simulink model "Dugoff0407"  (R2019a)
settings: Solver=VariableStepAuto  StartTime=0.0  StopTime=20  RelTol=1e-3
values from neighbouring files (symbols this model uses):
  a = 1.015    [Dugoff_parameter.m]
  b = 1.895    [Dugoff_parameter.m]
  g = 9.81    [Dugoff_parameter.m]
  hg = 0.54    [Dugoff_parameter.m]
  L = a+b    (= 2.91)    [Dugoff_parameter.m]
  ms = 1270    [Dugoff_parameter.m]
  mu = 0.85    [Dugoff_parameter.m]
  mw = 35.5    [Dugoff_parameter.m]
  R = 0.325    [Dugoff_parameter.m]
  tw1 = 1.675    [Dugoff_parameter.m]
  tw2 = 1.675    [Dugoff_parameter.m]
undefined symbols (not defined in the file or in its folder): Data, Data_SL_Info
libraries: robotlib x4, Solver_SF x1, sharedTrackingLibrary x1
settings Model: Creator=qidengliang  LastModifiedBy=Administrator
settings DataIOCC: ReturnWorkspaceOutputs=off
settings DebuggingCC: ArithmeticOperatorsInVariantConditions=warning
settings SFSimCC: SimUseLocalCustomCode=off
settings RTWCC: RTWUseLocalCustomCode=off

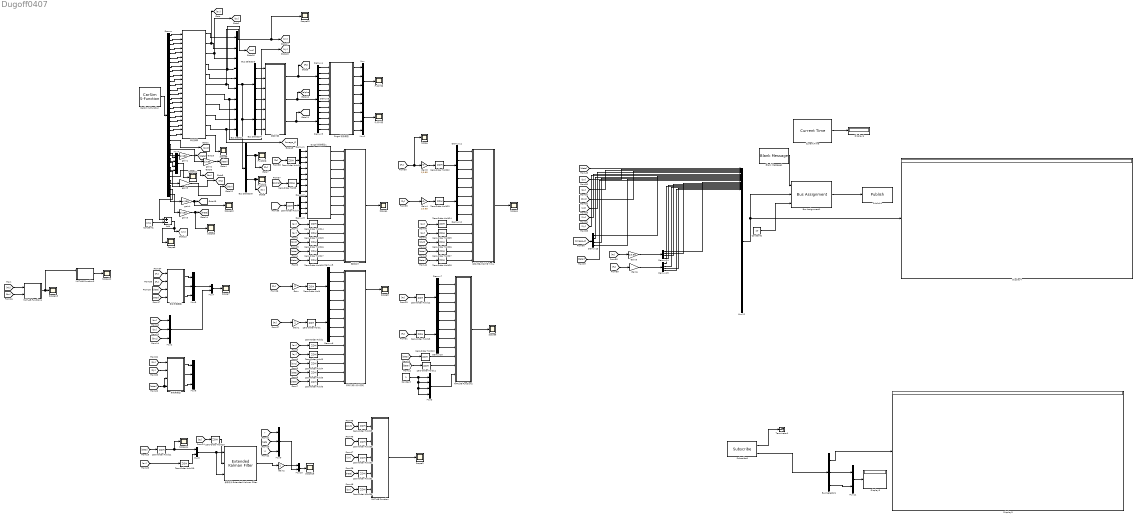
== system Dugoff0407 ==
  Add : Sum  Inputs=+-
  Blank Message1 : robotlib/Blank Message  messageClass=Message  entityType=std_msgs/Float64MultiArray  messageType=std_msgs/Float64MultiArray  SampleTime=-1
      settings: SourceProductBaseCode=RO
  Bus Assignment1 : BusAssignment  AssignedSignals=Data,Data_SL_Info.CurrentLength
  Bus Creator : BusCreator  Inputs=10
  Bus Selector1 : BusSelector  OutputSignals=Data,Data_SL_Info.CurrentLength,Data_SL_Info.ReceivedLength
  Bus Selector3 : BusSelector  OutputSignals=delta,ax,ay,omega
  Bus Selector4 : BusSelector  OutputSignals=Vx,Vy,r
  Bus Selector5 : BusSelector  OutputSignals=Fx,Fy
  CarSim S-Function : Solver_SF/CarSim S-Function  Priority=1  SIMFILE=simfile.sim
  Constant : Constant
  Constant1 : Constant  Value=0.54
  Constant2 : Constant  Value=20  OutDataTypeStr=uint32
  Current Time : robotlib/Current Time  OutputFormat=double  SampleTime=-1  ModelName=Dugoff0407
      settings: SourceProductName=Robotics System Toolbox  SourceProductBaseCode=RO
  Demux : Demux  Outputs=36
  Demux{1..15} (15 alike) : Demux
  Display{3..6} (4 alike) : Display
      Display3 settings: Format=long_e  Decimation=5
      Display4 settings: Format=long_e  Decimation=5
  Dugoff轮胎模型 : Subsystem
  Dugoff轮胎模型1 : Subsystem
  Fx估计值 : Scope
  Fx实际值 : Scope
  Fy估计值 : Scope
  Fy实际值 : Scope
  Gain : Gain  Gain=2
  Gain1 : Gain  Gain=2
  Gain2 : Gain
  Gain{3..6} (4 alike) : Gain  Gain=1/0.85
  MATLAB Function : MATLAB Function  TreatAsAtomicUnit=on
  MATLAB Function2 : MATLAB Function  TreatAsAtomicUnit=on
  MATLAB Function3 : MATLAB Function  TreatAsAtomicUnit=on
  MATLAB Function4 : MATLAB Function  TreatAsAtomicUnit=on
  Mux{,1,3..4} (4 alike) : Mux
  Mux{7..8,10..11} (4 alike) : Mux  Inputs=2
  Mux12 : Mux  Inputs=128
  Mux{2,5..6,9} (4 alike) : Mux  Inputs=3
  Publish1 : robotlib/Publish  topicSource=Specify your own  topic=/chatter/matlab  messageType=std_msgs/Float64MultiArray  messageQueueLength=1
      settings: SourceProductBaseCode=RO
  Scope{,1..16} (17 alike) : Scope
  Subscribe1 : robotlib/Subscribe  topicSource=Select from ROS network  topic=/chatter/array0  messageType=std_msgs/Float64MultiArray  sampleTime=-1  messageQueueLength=1
      settings: SourceProductBaseCode=RO
  Terminator1 : Terminator
  Zero-Order Hold{,1..33} (34 alike) : ZeroOrderHold  SampleTime=0.01
  gain{1..4} (4 alike) : Gain  Gain=pi/180
  gain5 : Gain  Gain=9.80665
  修正车辆模型 : MATLAB Function  TreatAsAtomicUnit=on
  单位换算 : Subsystem
  单转角模型 : MATLAB Function  TreatAsAtomicUnit=on
  参数估计Extended Kalman Filter : sharedTrackingLibrary/Extended Kalman Filter  StateTransitionFcn=LinearState2_u  HasStateTransitionJacobianFcn=off  HasAdditiveProcessNoise=Additive  ProcessNoise=diag([1 1 1])  HasTimeVaryingProcessNoise=off  HasStateTransitionFcnExtraArgument=1  InitialState=[0,0,13.9]  InitialStateCovariance=0.1  MeasurementFcn1=Sensor_ax_u2  HasMeasurementJacobianFcn1=off  HasMeasurementEnablePort1=off  HasAdditiveMeasurementNoise1=Additive  MeasurementNoise1=50  HasTimeVaryingMeasurementNoise1=off  HasMeasurementFcnExtraArgument1=1  MeasurementFcn2=myMeasurementFcn  HasMeasurementJacobianFcn2=off  HasMeasurementEnablePort2=off  HasAdditiveMeasurementNoise2=Additive  MeasurementNoise2=1  HasTimeVaryingMeasurementNoise2=off  HasMeasurementFcnExtraArgument2=0  MeasurementFcn3=myMeasurementFcn  HasMeasurementJacobianFcn3=off  HasMeasurementEnablePort3=off  HasAdditiveMeasurementNoise3=Additive  MeasurementNoise3=1  HasTimeVaryingMeasurementNoise3=off  HasMeasurementFcnExtraArgument3=0  MeasurementFcn4=myMeasurementFcn  HasMeasurementJacobianFcn4=off  HasMeasurementEnablePort4=off  HasAdditiveMeasurementNoise4=Additive  MeasurementNoise4=1  HasTimeVaryingMeasurementNoise4=off  HasMeasurementFcnExtraArgument4=0  MeasurementFcn5=myMeasurementFcn  HasMeasurementJacobianFcn5=off  HasMeasurementEnablePort5=off  HasAdditiveMeasurementNoise5=Additive  MeasurementNoise5=1  HasTimeVaryingMeasurementNoise5=off  HasMeasurementFcnExtraArgument5=0  EnableMultirate=off  StateTransitionFcnSampleTime=1  MeasurementFcn1SampleTime=1  MeasurementFcn2SampleTime=1  MeasurementFcn3SampleTime=1  MeasurementFcn4SampleTime=1  MeasurementFcn5SampleTime=1  UseCurrentEstimator=on  OutputStateCovariance=off  DataType=double  SampleTime=0.01  NumberOfMeasurements=1
      settings: SourceProductBaseCode=CT,DR,TF,ID,LP,NV,AR,RO,RR,UV,VE
  参数计算 : Subsystem
  实际力输入估计单个miu : MATLAB Function  TreatAsAtomicUnit=on
  实际力输入估计四轮 : MATLAB Function  TreatAsAtomicUnit=on
  整体估计 : MATLAB Function  TreatAsAtomicUnit=on
  wires:
  Demux/5 -> 单位换算/5(In5)
  Bus Selector5/1 -> [Fx], Fx实际值/1  "<Fx>"
  Demux/2 -> 单位换算/2(In2)
  Bus Selector3/2 -> 参数计算/2(ax)  "<ax>"
  CarSim S-Function/1 -> Demux/1
  Demux/23 -> 单位换算/23(In23)
  单位换算/11(alpha) -> Scope9/1  "真实值"
  单位换算/6(纵向车速) -> Scope15/1, [Vx], Bus Creator/6  "Vx"
  Demux/16 -> 单位换算/16(In16)
  Bus Creator/1 -> Bus Selector5/1, Bus Selector4/1, Bus Selector3/1
  Demux/22 -> 单位换算/22(In22)
  Demux/20 -> 单位换算/20(In20)
  Demux/12 -> 单位换算/12(In12)
  Demux/7 -> 单位换算/7(In7)
  Demux/21 -> 单位换算/21(In21)
  Demux/14 -> 单位换算/14(In14)
  Demux/9 -> 单位换算/9(In9)
  Demux/11 -> 单位换算/11(In11)
  Bus Selector5/2 -> [Fy], Fy实际值/1  "<Fy>"
  Bus Selector4/3 -> 参数计算/7(r)  "<r>"
  单位换算/4(横摆角速度) -> [wz], Bus Creator/4  "r"
  单位换算/3(侧向加速度) -> Bus Creator/3, [ay]  "ay"
  Demux4/3 -> Dugoff轮胎模型/3(Fz21)
  Demux/15 -> 单位换算/15(In15)
  单位换算/9(Fy_ij) -> Bus Creator/9  "Fy"
  Demux/1 -> 单位换算/1(In1)
  Demux/17 -> 单位换算/17(In17)
  单位换算/10(Omega_ij) -> [omega_ij], Bus Creator/10  "omega"
  单位换算/5(质心侧偏角) -> Bus Creator/5  "beta"
  Demux8/4 -> Dugoff轮胎模型/8(alpha22)
  Demux8/2 -> Dugoff轮胎模型/6(alpha12)
  Demux/8 -> 单位换算/8(In8)
  Bus Selector3/1 -> 参数计算/1(delta)  "<delta>"
  Demux/10 -> 单位换算/10(In10)
  Demux9/1 -> Dugoff轮胎模型/9(lamda11)
  Demux4/2 -> Dugoff轮胎模型/2(Fz12)
  Demux/18 -> 单位换算/18(In18)
  Demux/6 -> 单位换算/6(In6)
  单位换算/7(侧向车速) -> [Vy], Bus Creator/7  "Vy"
  Demux4/4 -> Dugoff轮胎模型/4(Fz22)
  Demux9/2 -> Dugoff轮胎模型/10(lamda12)
  Demux9/3 -> Dugoff轮胎模型/11(lamda21)
  Bus Selector3/3 -> 参数计算/3(ay)  "<ay>"
  Demux4/1 -> Dugoff轮胎模型/1(Fz11)
  Demux/13 -> 单位换算/13(In13)
  Demux9/4 -> Dugoff轮胎模型/12(lamda22)
  单位换算/2(纵向加速度) -> Bus Creator/2, [ax]  "ax"
  Demux8/3 -> Dugoff轮胎模型/7(alpha21)
  单位换算/8(Fx_ij) -> Bus Creator/8  "Fx"
  Demux8/1 -> Dugoff轮胎模型/5(alpha11)
  Bus Selector4/2 -> 参数计算/6(Vy)  "<Vy>"
  Demux/4 -> 单位换算/4(In4)
  Demux/19 -> 单位换算/19(In19)
  单位换算/1(前轮转角) -> Bus Creator/1  "delta"
  Bus Selector4/1 -> 参数计算/5(Vx)  "<Vx>"
  Demux/3 -> 单位换算/3(In3)
  Bus Selector3/4 -> 参数计算/4(omega)  "<omega>"
  Dugoff轮胎模型/3(Fx21) -> Mux/3
  Dugoff轮胎模型/2(Fx12) -> Mux/2
  Dugoff轮胎模型/1(Fx11) -> Mux/1
  Dugoff轮胎模型/4(Fx22) -> Mux/4
  Dugoff轮胎模型/5(Fy11) -> Mux1/1
  Dugoff轮胎模型/6(Fy12) -> Mux1/2
  Dugoff轮胎模型/7(Fy21) -> Mux1/3
  Dugoff轮胎模型/8(Fy22) -> Mux1/4
  Mux1/1 -> Fy估计值/1
  Mux/1 -> Fx估计值/1
  参数计算/1(Fz) -> [Fz], Demux4/1  "计算值"
  Demux1/1 -> Dugoff轮胎模型1/1(Fz11)
  Demux1/4 -> Dugoff轮胎模型1/4(Fz22)
  Demux1/2 -> Dugoff轮胎模型1/2(Fz12)
  Demux1/3 -> Dugoff轮胎模型1/3(Fz21)
  参数计算/2(alpha) -> [alpha], Demux8/1  "计算值"
  Demux2/1 -> Dugoff轮胎模型1/5(alpha11)
  Demux2/3 -> Dugoff轮胎模型1/7(alpha21)
  Demux3/4 -> Dugoff轮胎模型1/12(lamda22)
  Demux3/3 -> Dugoff轮胎模型1/11(lamda21)
  Demux3/2 -> Dugoff轮胎模型1/10(lamda12)
  Demux3/1 -> Dugoff轮胎模型1/9(lamda11)
  Demux2/2 -> Dugoff轮胎模型1/6(alpha12)
  Demux2/4 -> Dugoff轮胎模型1/8(alpha22)
  参数计算/3(lamda) -> [lamda], Demux9/1
  Dugoff轮胎模型1/8(Fy22) -> 整体估计/8(Fyrr)
  Dugoff轮胎模型1/7(Fy21) -> 整体估计/7(Fyrl)
  Dugoff轮胎模型1/6(Fy12) -> 整体估计/6(Fyfr)
  Dugoff轮胎模型1/5(Fy11) -> 整体估计/5(Fyfl)
  Dugoff轮胎模型1/4(Fx22) -> 整体估计/4(Fxrr)
  Dugoff轮胎模型1/3(Fx21) -> 整体估计/3(Fxrl)
  Dugoff轮胎模型1/2(Fx12) -> 整体估计/2(Fxfr)
  Dugoff轮胎模型1/1(Fx11) -> 整体估计/1(Fxfl)
  整体估计/1(x0) -> Scope4/1
  Demux/24 -> [dwz]
  gain1/1 -> [deta]
  Demux/25 -> gain1/1
  gain2/1 -> [detar]
  Demux/26 -> gain2/1
  实际力输入估计四轮/1(x0) -> Scope5/1
  Demux5/1 -> 实际力输入估计四轮/1(Fxfl)
  Demux5/2 -> 实际力输入估计四轮/2(Fxfr)
  Demux5/3 -> 实际力输入估计四轮/3(Fxrl)
  Demux5/4 -> 实际力输入估计四轮/4(Fxrr)
  Demux6/1 -> 实际力输入估计四轮/5(Fyfl)
  Demux6/2 -> 实际力输入估计四轮/6(Fyfr)
  Demux6/3 -> 实际力输入估计四轮/7(Fyrl)
  Demux6/4 -> 实际力输入估计四轮/8(Fyrr)
  Gain/1 -> Zero-Order Hold/1
  Gain1/1 -> Zero-Order Hold1/1
  Zero-Order Hold2/1 -> 实际力输入估计四轮/9(ax)
  Zero-Order Hold3/1 -> 实际力输入估计四轮/10(ay)
  Zero-Order Hold4/1 -> 实际力输入估计四轮/11(dwz)
  Zero-Order Hold5/1 -> 实际力输入估计四轮/12(deta)
  Zero-Order Hold6/1 -> 实际力输入估计四轮/13(detar)
  [detar] -> Zero-Order Hold6/1
  [deta] -> Zero-Order Hold5/1
  [ay] -> Zero-Order Hold3/1
  [dwz] -> Zero-Order Hold4/1
  [ax] -> Zero-Order Hold2/1
  [deta] -> Zero-Order Hold10/1
  [detar] -> Zero-Order Hold11/1
  Zero-Order Hold11/1 -> MATLAB Function2/10(detar)
  Zero-Order Hold10/1 -> MATLAB Function2/9(deta)
  Zero-Order Hold13/1 -> Demux10/1
  Zero-Order Hold12/1 -> Demux7/1
  Demux10/4 -> MATLAB Function2/8(Fyrr)
  Demux10/3 -> MATLAB Function2/7(Fyrl)
  Demux10/2 -> MATLAB Function2/6(Fyfr)
  Demux10/1 -> MATLAB Function2/5(Fyfl)
  Demux7/4 -> MATLAB Function2/4(Fxrr)
  Demux7/3 -> MATLAB Function2/3(Fxrl)
  Demux7/2 -> MATLAB Function2/2(Fxfr)
  Zero-Order Hold1/1 -> Demux6/1  "<Fy>"
  Zero-Order Hold/1 -> Demux5/1  "<Fx>"
  MATLAB Function2/1(zjian) -> Scope6/1
  [ax] -> Mux2/1
  [dwz] -> Mux2/3
  [ay] -> Mux2/2
  Constant/1 -> Mux3/4, Mux3/3, Mux3/2, Mux3/1
  Mux3/1 -> MATLAB Function2/11(x0)
  Zero-Order Hold7/1 -> Demux3/1
  Zero-Order Hold8/1 -> Demux2/1
  Zero-Order Hold9/1 -> Demux1/1
  [ax] -> Zero-Order Hold14/1
  [dwz] -> Zero-Order Hold16/1
  [ay] -> Zero-Order Hold15/1
  [deta] -> Zero-Order Hold17/1
  [detar] -> Zero-Order Hold18/1
  Zero-Order Hold18/1 -> 整体估计/13(detar)
  Zero-Order Hold17/1 -> 整体估计/12(deta)
  Zero-Order Hold16/1 -> 整体估计/11(dwz)
  Zero-Order Hold15/1 -> 整体估计/10(ay)
  Zero-Order Hold14/1 -> 整体估计/9(ax)
  Demux/27 -> Mux4/1
  Demux/28 -> Mux4/2
  Demux/29 -> Mux4/3
  Demux/30 -> Mux4/4
  Mux4/1 -> Scope11/1
  MATLAB Function3/1(y) -> Scope12/1
  Demux7/1 -> MATLAB Function2/1(Fxfl)
  Demux/31 -> [Tb]
  Demux/32 -> [dw]
  [Tb] -> MATLAB Function4/1(Tb)
  [dw] -> MATLAB Function4/2(dw)
  MATLAB Function4/1(y) -> MATLAB Function3/1(Fx), Scope13/1
  [deta] -> 修正车辆模型/3(detal)
  [detar] -> 修正车辆模型/4(detar)
  修正车辆模型/1(ax) -> Mux5/1
  修正车辆模型/3(dwz) -> Mux5/3
  [deta] -> 单转角模型/3(detal), 单转角模型/4(detar)
  单转角模型/3(dwz) -> Mux6/3
  单转角模型/2(ay) -> Mux6/2
  单转角模型/1(ax) -> Mux6/1
  修正车辆模型/2(ay) -> Mux5/2
  参数估计Extended Kalman Filter/1 -> Gain2/1
  Mux8/1 -> 参数估计Extended Kalman Filter/3, 参数估计Extended Kalman Filter/1
  Zero-Order Hold20/1 -> 参数估计Extended Kalman Filter/2
  Zero-Order Hold19/1 -> Mux8/2
  Zero-Order Hold21/1 -> Scope14/1, Mux8/1
  [deta] -> Zero-Order Hold21/1
  [beta] -> Mux9/2
  [r] -> Mux9/1
  [vx] -> Mux9/3
  Mux9/1 -> Mux10/2
  Gain2/1 -> Mux10/1
  Mux10/1 -> Scope16/1
  [ay] -> Zero-Order Hold20/1
  Mux5/1 -> Mux7/1
  Mux2/1 -> Mux7/2
  Mux7/1 -> Scope7/1
  [ax] -> Zero-Order Hold19/1
  [Fx] -> Gain/1
  [Fy] -> Gain1/1
  [Fx] -> Zero-Order Hold12/1
  [Fy] -> Zero-Order Hold13/1
  [Fx] -> 单转角模型/1(Fx)
  [Fy] -> 单转角模型/2(Fy)
  [Fy] -> 修正车辆模型/2(Fy)
  [Fx] -> 修正车辆模型/1(Fx)
  [lamda] -> Zero-Order Hold7/1
  [alpha] -> Zero-Order Hold8/1
  [Fz] -> Zero-Order Hold9/1
  [Fy] -> Gain4/1
  [Fx] -> Scope/1, Gain3/1
  Zero-Order Hold22/1 -> Demux11/1
  Zero-Order Hold23/1 -> Demux12/1
  [ax] -> Zero-Order Hold24/1
  [dwz] -> Zero-Order Hold26/1
  [ay] -> Zero-Order Hold25/1
  [deta] -> Zero-Order Hold27/1
  [detar] -> Zero-Order Hold28/1
  Zero-Order Hold28/1 -> 实际力输入估计单个miu/13(detar)
  Zero-Order Hold27/1 -> 实际力输入估计单个miu/12(deta)
  Zero-Order Hold26/1 -> 实际力输入估计单个miu/11(dwz)
  Zero-Order Hold25/1 -> 实际力输入估计单个miu/10(ay)
  Zero-Order Hold24/1 -> 实际力输入估计单个miu/9(ax)
  Gain4/1 -> Zero-Order Hold23/1
  Gain3/1 -> Zero-Order Hold22/1
  Demux12/4 -> 实际力输入估计单个miu/8(Fyrr)
  Demux12/3 -> 实际力输入估计单个miu/7(Fyrl)
  Demux12/2 -> 实际力输入估计单个miu/6(Fyfr)
  Demux12/1 -> 实际力输入估计单个miu/5(Fyfl)
  Demux11/4 -> 实际力输入估计单个miu/4(Fxrr)
  Demux11/3 -> 实际力输入估计单个miu/3(Fxrl)
  Demux11/2 -> 实际力输入估计单个miu/2(Fxfr)
  Demux11/1 -> 实际力输入估计单个miu/1(Fxfl)
  实际力输入估计单个miu/1(x0) -> Scope1/1
  gain3/1 -> Scope3/1, [theta]
  Demux/36 -> gain3/1
  Demux/34 -> gain4/1
  gain4/1 -> Scope10/1, [dtheta]
  gain5/1 -> [ddxh]
  Demux/33 -> gain5/1
  [theta] -> Zero-Order Hold32/1
  [ddxh] -> Zero-Order Hold29/1
  [dtheta] -> Zero-Order Hold30/1
  [xh] -> Zero-Order Hold31/1
  [ax] -> Zero-Order Hold33/1
  MATLAB Function/1(x0) -> Scope2/1
  Zero-Order Hold29/1 -> MATLAB Function/1(ddxh)
  Zero-Order Hold30/1 -> MATLAB Function/2(dtheta)
  Zero-Order Hold31/1 -> MATLAB Function/3(xh)
  Zero-Order Hold32/1 -> MATLAB Function/4(theta)
  Zero-Order Hold33/1 -> MATLAB Function/5(ax)
  Demux/35 -> Add/1
  Constant1/1 -> Add/2
  Add/1 -> Scope8/1, [xh]
  Demux14/4 -> Mux12/16
  Bus Selector1/1 -> Display3/1  "<Data>"
  Mux11/1 -> Display5/1
  Demux15/4 -> Mux12/20
  Subscribe1/1 -> Terminator1/1
  Gain6/1 -> Demux15/1
  [Fx] -> Gain5/1
  [Fy] -> Gain6/1
  [deta] -> Mux12/1  "delta"
  Bus Selector1/2 -> Mux11/1  "<CurrentLength>"
  Subscribe1/2 -> Bus Selector1/1
  Constant2/1 -> Bus Assignment1/3
  [wz] -> Mux12/5  "wz"
  Demux14/2 -> Mux12/14
  Demux15/1 -> Mux12/17
  Demux15/2 -> Mux12/18
  Current Time/1 -> Display6/1
  Demux15/3 -> Mux12/19
  Demux13/4 -> Mux12/11
  Demux13/2 -> Mux12/9
  Demux14/1 -> Mux12/13
  [Vy] -> Mux12/7  "Vy"
  Gain5/1 -> Demux14/1
  [detar] -> Mux12/12  "deltar"
  Bus Selector1/3 -> Mux11/2  "<ReceivedLength>"
  Demux14/3 -> Mux12/15
  [dwz] -> Mux12/4  "dwz"
  [Vx] -> Mux12/6  "Vx"
  Blank Message1/1 -> Bus Assignment1/1
  Demux13/3 -> Mux12/10
  [ax] -> Mux12/2  "ax"
  Demux13/1 -> Mux12/8
  Bus Assignment1/1 -> Publish1/1
  [omega_ij] -> Demux13/1
  Mux12/1 -> Display4/1, Bus Assignment1/2
  [ay] -> Mux12/3  "ay"

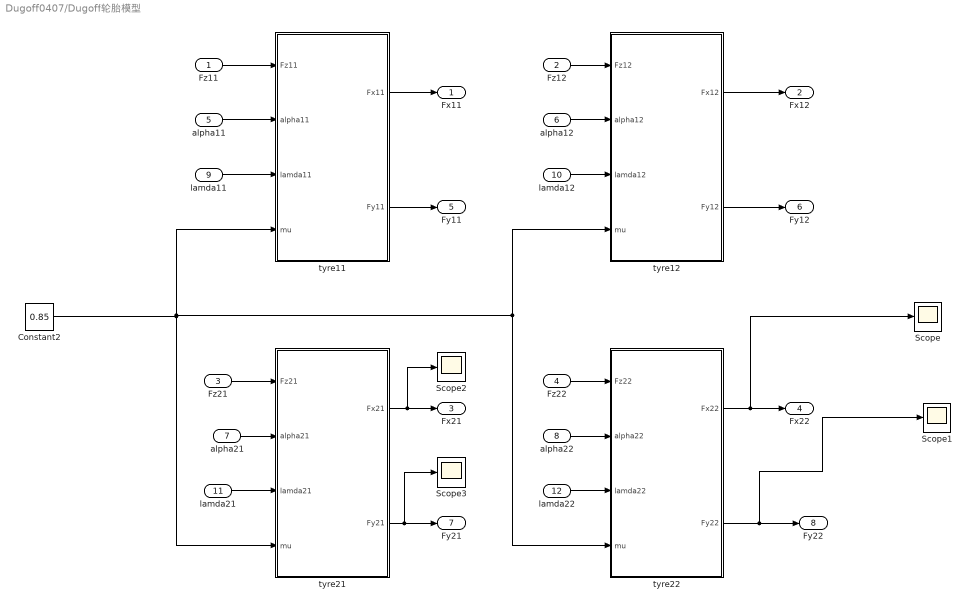
== system Dugoff0407/Dugoff轮胎模型 ==
  Fz11 : Inport
  Fz12 : Inport  Port=2
  Fz21 : Inport  Port=3
  Fz22 : Inport  Port=4
  alpha11 : Inport  Port=5
  alpha12 : Inport  Port=6
  alpha21 : Inport  Port=7
  alpha22 : Inport  Port=8
  lamda11 : Inport  Port=9
  lamda12 : Inport  Port=10
  lamda21 : Inport  Port=11
  lamda22 : Inport  Port=12
  Constant2 : Constant  Value=0.85
  Scope{,1..3} (4 alike) : Scope
  tyre11 : MATLAB Function  TreatAsAtomicUnit=on
  tyre12 : MATLAB Function  TreatAsAtomicUnit=on
  tyre21 : MATLAB Function  TreatAsAtomicUnit=on
  tyre22 : MATLAB Function  TreatAsAtomicUnit=on
  Fx11 : Outport
  Fx12 : Outport  Port=2
  Fx21 : Outport  Port=3
  Fx22 : Outport  Port=4
  Fy11 : Outport  Port=5
  Fy12 : Outport  Port=6
  Fy21 : Outport  Port=7
  Fy22 : Outport  Port=8
  wires:
  Constant2/1 -> tyre11/4(mu), tyre22/4(mu), tyre12/4(mu), tyre21/4(mu)
  alpha21/1 -> tyre21/2(alpha21)
  tyre22/2(Fy22) -> Scope1/1, Fy22/1
  Fz12/1 -> tyre12/1(Fz12)
  Fz21/1 -> tyre21/1(Fz21)
  tyre21/2(Fy21) -> Scope3/1, Fy21/1
  tyre12/2(Fy12) -> Fy12/1
  lamda12/1 -> tyre12/3(lamda12)
  tyre11/1(Fx11) -> Fx11/1
  tyre12/1(Fx12) -> Fx12/1
  tyre22/1(Fx22) -> Scope/1, Fx22/1
  lamda22/1 -> tyre22/3(lamda22)
  alpha12/1 -> tyre12/2(alpha12)
  Fz11/1 -> tyre11/1(Fz11)
  alpha11/1 -> tyre11/2(alpha11)
  lamda21/1 -> tyre21/3(lamda21)
  lamda11/1 -> tyre11/3(lamda11)
  Fz22/1 -> tyre22/1(Fz22)
  alpha22/1 -> tyre22/2(alpha22)
  tyre11/2(Fy11) -> Fy11/1
  tyre21/1(Fx21) -> Scope2/1, Fx21/1

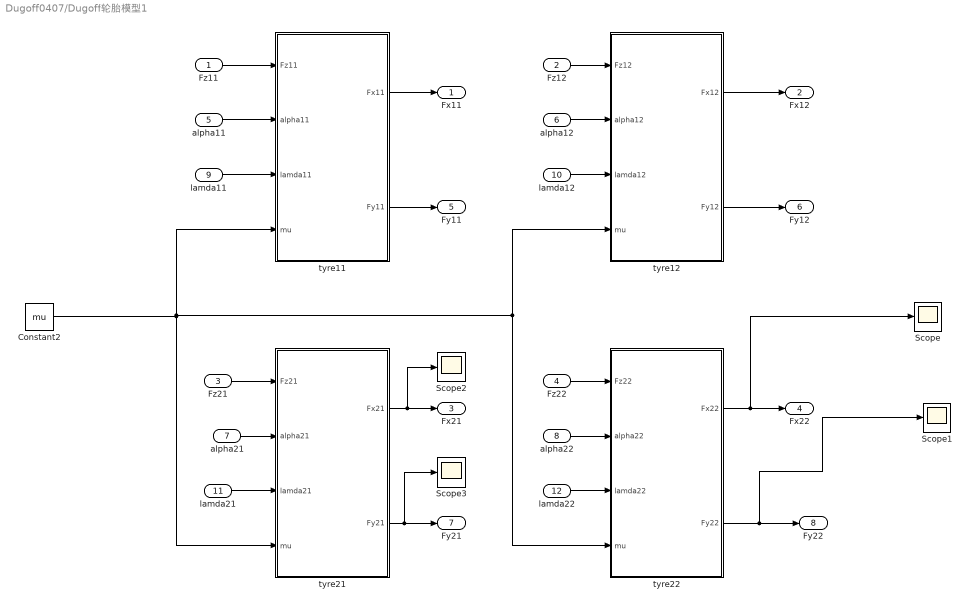
== system Dugoff0407/Dugoff轮胎模型1 ==
  Fz11 : Inport
  Fz12 : Inport  Port=2
  Fz21 : Inport  Port=3
  Fz22 : Inport  Port=4
  alpha11 : Inport  Port=5
  alpha12 : Inport  Port=6
  alpha21 : Inport  Port=7
  alpha22 : Inport  Port=8
  lamda11 : Inport  Port=9
  lamda12 : Inport  Port=10
  lamda21 : Inport  Port=11
  lamda22 : Inport  Port=12
  Constant2 : Constant  Value=mu
  Scope{,1..3} (4 alike) : Scope
  tyre11 : MATLAB Function  TreatAsAtomicUnit=on
  tyre12 : MATLAB Function  TreatAsAtomicUnit=on
  tyre21 : MATLAB Function  TreatAsAtomicUnit=on
  tyre22 : MATLAB Function  TreatAsAtomicUnit=on
  Fx11 : Outport
  Fx12 : Outport  Port=2
  Fx21 : Outport  Port=3
  Fx22 : Outport  Port=4
  Fy11 : Outport  Port=5
  Fy12 : Outport  Port=6
  Fy21 : Outport  Port=7
  Fy22 : Outport  Port=8
  wires:
  tyre21/1(Fx21) -> Fx21/1, Scope2/1
  tyre11/2(Fy11) -> Fy11/1
  alpha22/1 -> tyre22/2(alpha22)
  Fz22/1 -> tyre22/1(Fz22)
  lamda11/1 -> tyre11/3(lamda11)
  lamda21/1 -> tyre21/3(lamda21)
  alpha11/1 -> tyre11/2(alpha11)
  Fz11/1 -> tyre11/1(Fz11)
  alpha12/1 -> tyre12/2(alpha12)
  lamda22/1 -> tyre22/3(lamda22)
  tyre22/1(Fx22) -> Fx22/1, Scope/1
  tyre12/1(Fx12) -> Fx12/1
  tyre11/1(Fx11) -> Fx11/1
  lamda12/1 -> tyre12/3(lamda12)
  tyre12/2(Fy12) -> Fy12/1
  tyre21/2(Fy21) -> Fy21/1, Scope3/1
  Fz21/1 -> tyre21/1(Fz21)
  Fz12/1 -> tyre12/1(Fz12)
  tyre22/2(Fy22) -> Fy22/1, Scope1/1
  alpha21/1 -> tyre21/2(alpha21)
  Constant2/1 -> tyre21/4(mu), tyre12/4(mu), tyre22/4(mu), tyre11/4(mu)

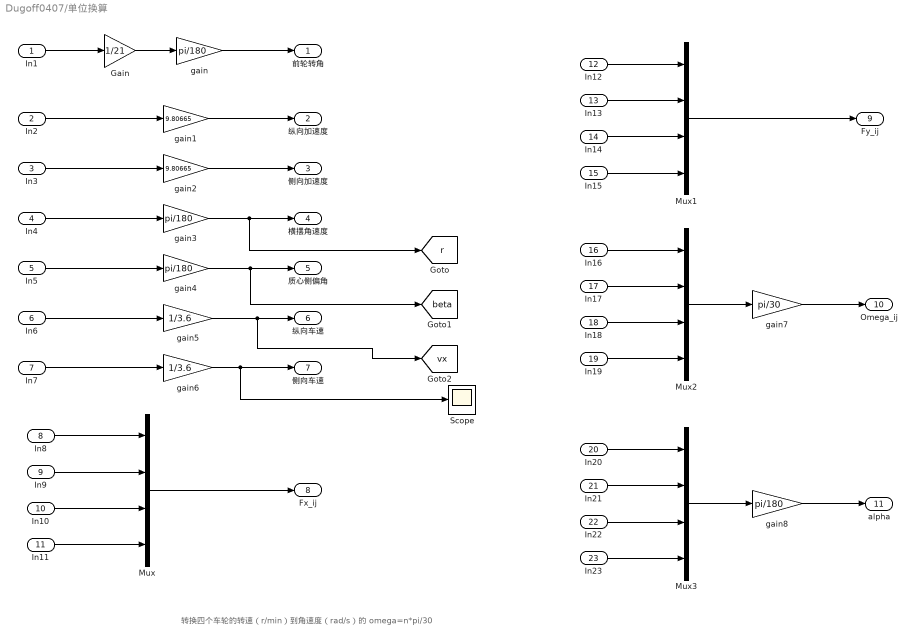
== system Dugoff0407/单位换算 ==
  note: 转换四个车轮的转速（r/min）到角速度（rad/s）的
      | omega=n*pi/30
  In1 : Inport
  In2 : Inport  Port=2
  In3 : Inport  Port=3
  In4 : Inport  Port=4
  In5 : Inport  Port=5
  In6 : Inport  Port=6
  In7 : Inport  Port=7
  In8 : Inport  Port=8
  In9 : Inport  Port=9
  In10 : Inport  Port=10
  In11 : Inport  Port=11
  In12 : Inport  Port=12
  In13 : Inport  Port=13
  In14 : Inport  Port=14
  In15 : Inport  Port=15
  In16 : Inport  Port=16
  In17 : Inport  Port=17
  In18 : Inport  Port=18
  In19 : Inport  Port=19
  In20 : Inport  Port=20
  In21 : Inport  Port=21
  In22 : Inport  Port=22
  In23 : Inport  Port=23
  Gain : Gain  Gain=1/21
  Mux{,1..3} (4 alike) : Mux
  Scope : Scope
  gain{,3..4,8} (4 alike) : Gain  Gain=pi/180
  gain1 : Gain  Gain=9.80665
  gain2 : Gain  Gain=9.80665
  gain5 : Gain  Gain=1/3.6
  gain6 : Gain  Gain=1/3.6
  gain7 : Gain  Gain=pi/30
  前轮转角 : Outport
  纵向加速度 : Outport  Port=2
  侧向加速度 : Outport  Port=3
  横摆角速度 : Outport  Port=4
  质心侧偏角 : Outport  Port=5
  纵向车速 : Outport  Port=6
  侧向车速 : Outport  Port=7
  Fx_ij : Outport  Port=8
  Fy_ij : Outport  Port=9
  Omega_ij : Outport  Port=10
  alpha : Outport  Port=11
  tag scope: beta=global, r=global, vx=global
  wires:
  In8/1 -> Mux/1
  In10/1 -> Mux/3
  In1/1 -> Gain/1
  In15/1 -> Mux1/4
  In9/1 -> Mux/2
  In11/1 -> Mux/4
  Mux/1 -> Fx_ij/1
  In14/1 -> Mux1/3
  In12/1 -> Mux1/1
  In13/1 -> Mux1/2
  gain/1 -> 前轮转角/1
  In2/1 -> gain1/1
  In3/1 -> gain2/1
  In4/1 -> gain3/1
  In5/1 -> gain4/1
  In6/1 -> gain5/1
  In7/1 -> gain6/1
  gain1/1 -> 纵向加速度/1
  gain2/1 -> 侧向加速度/1
  gain3/1 -> [r], 横摆角速度/1
  gain4/1 -> [beta], 质心侧偏角/1
  gain5/1 -> [vx], 纵向车速/1
  gain6/1 -> Scope/1, 侧向车速/1
  Gain/1 -> gain/1
  Mux1/1 -> Fy_ij/1
  gain7/1 -> Omega_ij/1
  Mux2/1 -> gain7/1
  In16/1 -> Mux2/1
  In17/1 -> Mux2/2
  In18/1 -> Mux2/3
  In19/1 -> Mux2/4
  In21/1 -> Mux3/2
  In22/1 -> Mux3/3
  In20/1 -> Mux3/1
  In23/1 -> Mux3/4
  Mux3/1 -> gain8/1
  gain8/1 -> alpha/1

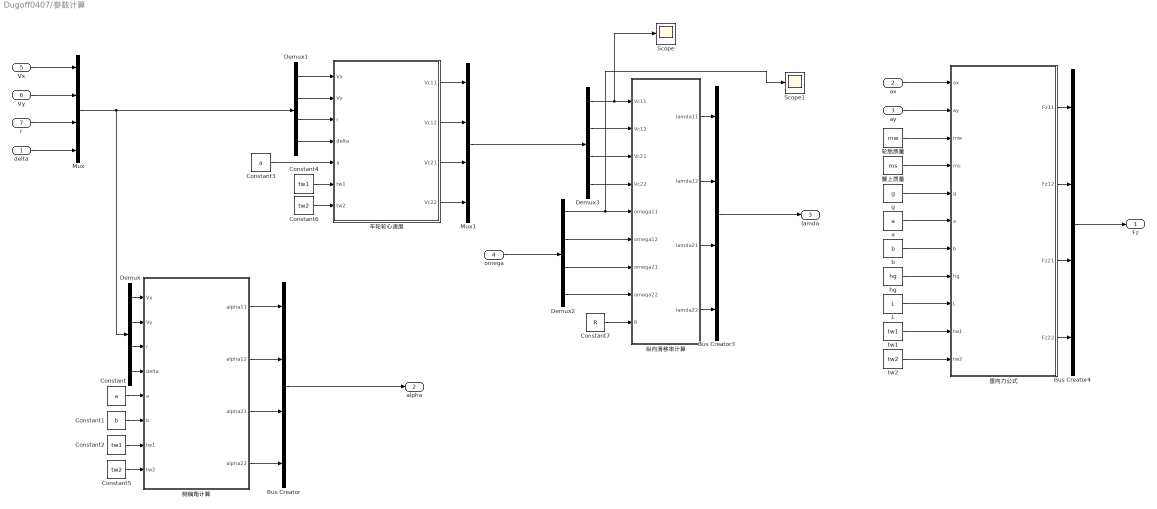
== system Dugoff0407/参数计算 ==
  delta : Inport
  ax : Inport  Port=2
  ay : Inport  Port=3
  omega : Inport  Port=4
  Vx : Inport  Port=5
  Vy : Inport  Port=6
  r : Inport  Port=7
  Bus Creator : BusCreator  Inputs=4
  Bus Creator3 : BusCreator  Inputs=4
  Bus Creator4 : BusCreator  Inputs=4
  Constant : Constant  Value=a
  Constant1 : Constant  Value=b
  Constant2 : Constant  Value=tw1
  Constant3 : Constant  Value=a
  Constant4 : Constant  Value=tw1
  Constant5 : Constant  Value=tw2
  Constant6 : Constant  Value=tw2
  Constant7 : Constant  Value=R
  Demux{,1..3} (4 alike) : Demux
  L : Constant  Value=L
  Mux : Mux
  Mux1 : Mux
  Scope : Scope
  Scope1 : Scope
  a : Constant  Value=a
  b : Constant  Value=b
  g : Constant  Value=g
  hg : Constant  Value=hg
  tw1 : Constant  Value=tw1
  tw2 : Constant  Value=tw2
  侧偏角计算 : MATLAB Function  TreatAsAtomicUnit=on
  垂向力公式 : MATLAB Function  TreatAsAtomicUnit=on
  簧上质量 : Constant  Value=ms
  纵向滑移率计算 : MATLAB Function  TreatAsAtomicUnit=on
  车轮轮心速度 : MATLAB Function  TreatAsAtomicUnit=on
  轮胎质量 : Constant  Value=mw
  Fz : Outport
  alpha : Outport  Port=2
  lamda : Outport  Port=3
  wires:
  Demux/1 -> 侧偏角计算/1(Vx)
  垂向力公式/2(Fz12) -> Bus Creator4/2
  垂向力公式/3(Fz21) -> Bus Creator4/3
  纵向滑移率计算/1(lamda11) -> Bus Creator3/1
  纵向滑移率计算/2(lamda12) -> Bus Creator3/2
  轮胎质量/1 -> 垂向力公式/3(mw)
  hg/1 -> 垂向力公式/8(hg)
  Demux2/3 -> 纵向滑移率计算/7(omega21)
  Demux/3 -> 侧偏角计算/3(r)
  g/1 -> 垂向力公式/5(g)
  Demux2/2 -> 纵向滑移率计算/6(omega12)
  tw1/1 -> 垂向力公式/10(tw1)
  纵向滑移率计算/3(lamda21) -> Bus Creator3/3
  垂向力公式/1(Fz11) -> Bus Creator4/1
  Demux1/3 -> 车轮轮心速度/3(r)
  Constant/1 -> 侧偏角计算/5(a)
  Demux/2 -> 侧偏角计算/2(Vy)
  Constant4/1 -> 车轮轮心速度/6(tw1)
  Demux2/1 -> Scope1/1, 纵向滑移率计算/5(omega11)
  Constant3/1 -> 车轮轮心速度/5(a)
  Demux1/4 -> 车轮轮心速度/4(delta)
  L/1 -> 垂向力公式/9(L)
  Demux1/2 -> 车轮轮心速度/2(Vy)
  Demux2/4 -> 纵向滑移率计算/8(omega22)
  垂向力公式/4(Fz22) -> Bus Creator4/4
  Constant2/1 -> 侧偏角计算/7(tw1)
  a/1 -> 垂向力公式/6(a)
  Demux1/1 -> 车轮轮心速度/1(Vx)
  Constant1/1 -> 侧偏角计算/6(b)
  纵向滑移率计算/4(lamda22) -> Bus Creator3/4
  Demux/4 -> 侧偏角计算/4(delta)
  Constant7/1 -> 纵向滑移率计算/9(R)
  侧偏角计算/1(alpha11) -> Bus Creator/1
  b/1 -> 垂向力公式/7(b)
  Bus Creator4/1 -> Fz/1
  Bus Creator3/1 -> lamda/1
  tw2/1 -> 垂向力公式/11(tw2)
  Constant5/1 -> 侧偏角计算/8(tw2)
  Constant6/1 -> 车轮轮心速度/7(tw2)
  delta/1 -> Mux/4
  ax/1 -> 垂向力公式/1(ax)
  ay/1 -> 垂向力公式/2(ay)
  Vy/1 -> Mux/2
  Vx/1 -> Mux/1
  Mux/1 -> Demux/1, Demux1/1
  车轮轮心速度/1(Vc11) -> Mux1/1
  车轮轮心速度/2(Vc12) -> Mux1/2
  车轮轮心速度/3(Vc21) -> Mux1/3
  车轮轮心速度/4(Vc22) -> Mux1/4
  Demux3/1 -> Scope/1, 纵向滑移率计算/1(Vc11)
  Demux3/2 -> 纵向滑移率计算/2(Vc12)
  Demux3/3 -> 纵向滑移率计算/3(Vc21)
  Demux3/4 -> 纵向滑移率计算/4(Vc22)
  侧偏角计算/4(alpha22) -> Bus Creator/4
  侧偏角计算/3(alpha21) -> Bus Creator/3
  侧偏角计算/2(alpha12) -> Bus Creator/2
  Bus Creator/1 -> alpha/1
  簧上质量/1 -> 垂向力公式/4(ms)
  Mux1/1 -> Demux3/1
  r/1 -> Mux/3
  omega/1 -> Demux2/1

== matlab function Dugoff0407/Dugoff轮胎模型1/tyre11 ==
  data: Fx11 output; Fy11 output; Fz11 input; alpha11 input; lamda11 input; mu input
function [Fx11,Fy11] = fcn(Fz11,alpha11,lamda11,mu)
lamda11=-lamda11;

  Cx=-30; 
  Cy=-18;    

S=(1-lamda11)/(2*sqrt((Cx^2)*(lamda11^2)+(Cy^2)*(tan(alpha11))^2));
if S<1
   f=S*(2-S);
else            %S>=1
   f=1;
end


Fx11=Fz11*Cx*lamda11*f/(1-lamda11);
Fy11=Fz11*Cy*tan(alpha11)*f/(1-lamda11);
% 
%   Cx=-30; 
%   Cy=-18;

== matlab function Dugoff0407/整体估计 ==
  data: Fxfl input; x0 output; Fxfr input; Fxrl input; Fxrr input; Fyfl input; Fyfr input; Fyrl input; Fyrr input; ax input; ay input; dwz input; deta input; detar input
function x0 = fcn(Fxfl,Fxfr,Fxrl,Fxrr,Fyfl,Fyfr,Fyrl,Fyrr,ax,ay,dwz,deta,detar)
persistent X P;
if isempty(X)
    X = 0.6;
    P =0.001;
end

m=1412;
la=1.015; %质心距离前轴的距离m 1.27 
lb=1.895; %质心距离后轴的距离m
Tf=1.675; %前轴轮距m
Tr=1.675; %后轴轮距m 1.55
Iz=1536.7; %整车z轴转动惯量kg*m^2
Q = 0.001;
R = diag([1,1,1])*50;
Xpre = X;
%F = diag([1,1,1,1]);
H = [(Fxfl*cos(deta)-Fyfl*sin(deta))/m+(Fxfr*cos(detar)-Fyfr*sin(detar))/m+Fxrl/m+Fxrr/m;(Fxfl*sin(deta)+Fyfl*cos(deta))/m+(Fxfr*sin(detar)+Fyfr*cos(deta))/m+Fyrl/m+Fyrr/m;(la*(Fxfl*sin(deta)+Fyfl*cos(deta))-Tf/2*(Fxfl*cos(deta)-Fyfl*sin(deta)))/Iz+(la*(Fxfr*sin(detar)+Fyfr*cos(detar))+Tf/2*(Fxfr*cos(detar)-Fyfr*sin(detar)))/Iz+(-Tr/2*Fxrl-lb*Fyrl)/Iz+(Tr/2*Fxrr-lb*Fyrr)/Iz];
zjian =H*Xpre; 
PP=P+Q;
% if a>0
if (H*PP*H')~=zeros(3,3)

% if(det(H*PP*H'+R)==0)
%     X = ones(4, 1);
% else
Kk=PP*H'/(H*PP*H'+R);
X=Xpre+Kk*([ax,ay,dwz]'-zjian);
P=PP-Kk*H*PP;
% end
% 
% if(X(1)>1||X(1)<0||X(2)<0||X(3)<0||X(4)<0||X(2)>1||X(3)>1||X(4)>1)
%     X=0.8;
%     P=0.001;
% else
% end
x0=X;
else
    x0 = zeros(1,1);
    
end
% else
%     x0 = zeros(4,1);
%     X=ones(4, 1)*0.5;
%     P=diag([1,1,1,1])*0.1;
%     ccc = 2;
% end
end

== matlab function Dugoff0407/Dugoff轮胎模型1/tyre12 ==
  data: Fx12 output; Fy12 output; Fz12 input; alpha12 input; lamda12 input; mu input
function [Fx12,Fy12] = fcn(Fz12,alpha12,lamda12,mu)
lamda12=-lamda12;

 Cx=-28;
 Cy=-18.5;

S=(1-lamda12)/(2*sqrt(Cx^2*lamda12^2+Cy^2*(tan(alpha12))^2));
if S<1
   f=S*(2-S);
else
   f=1;
end
Fx12=Fz12*Cx*lamda12*f/(1-lamda12);
Fy12=Fz12*Cy*tan(alpha12)*f/(1-lamda12);


%  Cx=-28;
%  Cy=-18.5;

== matlab function Dugoff0407/Dugoff轮胎模型1/tyre21 ==
  data: Fx21 output; Fy21 output; Fz21 input; alpha21 input; lamda21 input; mu input
function [Fx21,Fy21] = fcn(Fz21,alpha21,lamda21,mu)
lamda21=-lamda21

  Cx=-30;
  Cy=-20.5;

S=(1-lamda21)/(2*sqrt((Cx^2)*(lamda21^2)+(Cy^2)*((tan(alpha21))^2)));
if S<1
   f=S*(2-S);
else
   f=1;
end
Fx21=Fz21*Cx*lamda21*f/(1-lamda21);
Fy21=Fz21*Cy*tan(alpha21)*f/(1-lamda21);

%   Cx=-30;
%   Cy=-20.5;

== matlab function Dugoff0407/Dugoff轮胎模型1/tyre22 ==
  data: Fx22 output; Fy22 output; Fz22 input; alpha22 input; lamda22 input; mu input
function [Fx22,Fy22] = fcn(Fz22,alpha22,lamda22,mu)
  lamda22=-lamda22
  
  Cx=-31;
  Cy=-20;

S=(1-lamda22)/(2*sqrt(Cx^2*lamda22^2+Cy^2*(tan(alpha22))^2));
if S<1
   f=S*(2-S);
else
   f=1;
end
Fx22=Fz22*Cx*lamda22*f/(1-lamda22);
Fy22=Fz22*Cy*tan(alpha22)*f/(1-lamda22);

%   Cx=-31;
%   Cy=-20;

== matlab function Dugoff0407/MATLAB Function2 ==
  data: Fxfl input; zjian output; Fxfr input; Fxrl input; Fxrr input; Fyfl input; Fyfr input; Fyrl input; Fyrr input; deta input; detar input; x0 input
function zjian = fcn(Fxfl,Fxfr,Fxrl,Fxrr,Fyfl,Fyfr,Fyrl,Fyrr,deta,detar,x0)

m=1412;
la=1.015; %质心距离前轴的距离m 1.27 
lb=1.895; %质心距离后轴的距离m
Tf=1.675; %前轴轮距m
Tr=1.675; %后轴轮距m 1.55
Iz=1536.7; %整车z轴转动惯量kg*m^2

Xpre = x0;
%F = diag([1,1,1,1]);
H = [(Fxfl*cos(deta)-Fyfl*sin(deta))/m,(Fxfr*cos(detar)-Fyfr*sin(detar))/m,Fxrl/m,Fxrr/m;(Fxfl*sin(deta)+Fyfl*cos(deta))/m,(Fxfr*sin(detar)+Fyfr*cos(detar))/m,Fyrl/m,Fyrr/m;(la*(Fxfl*sin(deta)+Fyfl*cos(deta))-Tf/2*(Fxfl*cos(deta)-Fyfl*sin(deta)))/Iz,(la*(Fxfr*sin(detar)+Fyfr*cos(detar))+Tf/2*(Fxfr*cos(detar)-Fyfr*sin(detar)))/Iz,(-Tr/2*Fxrl-lb*Fyrl)/Iz,(Tr/2*Fxrr-lb*Fyrr)/Iz];
zjian =H*Xpre; 

end

== matlab function Dugoff0407/MATLAB Function3 ==
  data: Fx input; y output; Fz input; lamda input
function y = fcn(Fx,Fz,lamda)


y = Fx/Fz/lamda;
end

== matlab function Dugoff0407/MATLAB Function4 ==
  data: Tb input; y output; dw input
function y = fcn(Tb,dw)
R=0.325;
y = (2*dw+Tb)/R;

== matlab function Dugoff0407/参数计算/侧偏角计算 ==
  data: Vx input; alpha11 output; alpha12 output; alpha21 output; alpha22 output; Vy input; r input; delta input; a input; b input; tw1 input; tw2 input
function [alpha11,alpha12,alpha21,alpha22] = fcn(Vx,Vy,r,delta,a,b,tw1,tw2)
a=0.72;  %对应的是carsim中的车速为40的时候
b=1.895;
% a=0.75;
% b=1.9;

alpha11= -delta+atan((Vy+a*r)/(Vx-tw1*r/2));
alpha12= -delta+atan((Vy+a*r)/(Vx+tw1*r/2));
alpha21=  atan((Vy-b*r)/(Vx-tw2*r/2));
alpha22=  atan((Vy-b*r)/(Vx+tw2*r/2));

== matlab function Dugoff0407/参数计算/垂向力公式 ==
  data: ax input; ay input; mw input; Fz11 output; Fz12 output; Fz21 output; Fz22 output; ms input; g input; a input; b input; hg input; L input; tw1 input; tw2 input
function [Fz11,Fz12,Fz21,Fz22] = fcn(ax,ay,mw,ms,g,a,b,hg,L,tw1,tw2)

Fz11=mw*g+ms*g*b/2/L-ms*hg*ax/2/L-ms*hg*ay/2/tw1;
Fz12=mw*g+ms*g*b/2/L-ms*hg*ax/2/L+ms*hg*ay/2/tw1;
Fz21=mw*g+ms*g*a/2/L+ms*hg*ax/2/L-ms*hg*ay/2/tw2;
Fz22=mw*g+ms*g*a/2/L+ms*hg*ax/2/L+ms*hg*ay/2/tw2;

== matlab function Dugoff0407/参数计算/纵向滑移率计算 ==
  data: Vc11 input; lamda11 output; lamda12 output; lamda21 output; lamda22 output; Vc12 input; Vc21 input; Vc22 input; omega11 input; omega12 input; omega21 input; omega22 input; R input
function [lamda11,lamda12,lamda21,lamda22] = fcn(Vc11,Vc12,Vc21,Vc22,omega11,omega12,omega21,omega22,R)

%R=0.325005;
lamda11=(omega11*R-Vc11)/Vc11;
lamda12=(omega12*R-Vc12)/Vc12;
lamda21=(omega21*R-Vc21)/Vc21;
lamda22=(omega22*R-Vc22)/Vc22;

== matlab function Dugoff0407/参数计算/车轮轮心速度 ==
  data: Vx input; Vc11 output; Vc12 output; Vc21 output; Vc22 output; Vy input; r input; delta input; a input; tw1 input; tw2 input
function [Vc11,Vc12,Vc21,Vc22] = fcn(Vx,Vy,r,delta,a,tw1,tw2)
Vc11=(Vx-tw1*r/2)*cos(delta)+(Vy+a*r)*sin(delta);
Vc12=(Vx+tw1*r/2)*cos(delta)+(Vy+a*r)*sin(delta);
Vc21=Vx-tw2*r/2;
Vc22=Vx+tw2*r/2;

== matlab function Dugoff0407/修正车辆模型 ==
  data: Fx input; ax output; Fy input; detal input; detar input; ay output; dwz output
function [ax,ay,dwz] = fcn(Fx,Fy,detal,detar)
m=1412;
Iz=1.536700000000000e+03;
Lf=1.015;
Lr=1.895;
Bf=1.675;
Br=1.675;
ax=(Fx(1)*cos(detal)-Fy(1)*sin(detal))/m+(Fx(2)*cos(detar)-Fy(2)*sin(detar))/m+Fx(3)/m+Fx(4)/m; 
ay=(Fx(1)*sin(detal)+Fy(1)*cos(detal))/m+(Fx(2)*sin(detar)+Fy(2)*cos(detar))/m+Fy(3)/m+Fy(4)/m;
dwz=(Lf*(Fx(1)*sin(detal)+Fy(1)*cos(detal))-0.5*Bf*(Fx(1)*cos(detal)-Fy(1)*sin(detal)))/Iz+(Lf*(Fx(2)*sin(detar)+Fy(2)*cos(detar))+0.5*Bf*(Fx(2)*cos(detar)-Fy(2)*sin(detar)))/Iz-(0.5*Br*Fx(3)+Lr*Fy(3))/Iz+(0.5*Br*Fx(4)-Lr*Fy(4))/Iz;
end

== matlab function Dugoff0407/实际力输入估计四轮 ==
  data: Fxfl input; x0 output; Fxfr input; Fxrl input; Fxrr input; Fyfl input; Fyfr input; Fyrl input; Fyrr input; ax input; ay input; dwz input; deta input; detar input; H output; ccc output
function [x0,H, ccc]= fcn(Fxfl,Fxfr,Fxrl,Fxrr,Fyfl,Fyfr,Fyrl,Fyrr,ax,ay,dwz,deta,detar)
persistent X P a;
if isempty(X)
    X = ones(4, 1)*0.6;
    P =diag([1,1,1,1])*0.001;
    a=0;
end

m=1412;
la=1.015; %质心距离前轴的距离m 1.27 
lb=1.895; %质心距离后轴的距离m
Tf=1.675; %前轴轮距m
Tr=1.675; %后轴轮距m 1.55
Iz=1536.7; %整车z轴转动惯量kg*m^2
Q = diag([1,1,1,1])*0.001;
R = diag([1,1,1])*50;
Xpre = X;
%F = diag([1,1,1,1]);
H = [(Fxfl*cos(deta)-Fyfl*sin(deta))/m,(Fxfr*cos(detar)-Fyfr*sin(detar))/m,Fxrl/m,Fxrr/m;(Fxfl*sin(deta)+Fyfl*cos(deta))/m,(Fxfr*sin(detar)+Fyfr*cos(deta))/m,Fyrl/m,Fyrr/m;(la*(Fxfl*sin(deta)+Fyfl*cos(deta))-Tf/2*(Fxfl*cos(deta)-Fyfl*sin(deta)))/Iz,(la*(Fxfr*sin(detar)+Fyfr*cos(detar))+Tf/2*(Fxfr*cos(detar)-Fyfr*sin(detar)))/Iz,(-Tr/2*Fxrl-lb*Fyrl)/Iz,(Tr/2*Fxrr-lb*Fyrr)/Iz];
zjian =H*Xpre; 
PP=P+Q;
a=a+1;
% if a>0
if (H*PP*H')~=zeros(3,3)

% if(det(H*PP*H'+R)==0)
%     X = ones(4, 1);
% else
Kk=PP*H'/(H*PP*H'+R);
X=Xpre+Kk*([ax,ay,dwz]'-zjian);
P=PP-Kk*H*PP;
% end

if(X(1)>1||X(1)<0||X(2)<0||X(3)<0||X(4)<0||X(2)>1||X(3)>1||X(4)>1)
    X=ones(4, 1)*0.6;
    P=diag([1,1,1,1])*0.001;
else
end
x0=X;
ccc = 0;
else
    x0 = zeros(4,1);
    ccc = 1;
    
end
% else
%     x0 = zeros(4,1);
%     X=ones(4, 1)*0.5;
%     P=diag([1,1,1,1])*0.1;
%     ccc = 2;
% end
end

== matlab function Dugoff0407/单转角模型 ==
  data: Fx input; ax output; Fy input; detal input; detar input; ay output; dwz output
function [ax,ay,dwz] = fcn(Fx,Fy,detal,detar)
m=1412;
Iz=1.536700000000000e+03;
Lf=1.015;
Lr=1.895;
Bf=1.675;
Br=1.675;
ax=(Fx(1)*cos(detal)-Fy(1)*sin(detal))/m+(Fx(2)*cos(detar)-Fy(2)*sin(detar))/m+Fx(3)/m+Fx(4)/m; 
ay=(Fx(1)*sin(detal)+Fy(1)*cos(detal))/m+(Fx(2)*sin(detar)+Fy(2)*cos(detar))/m+Fy(3)/m+Fy(4)/m;
dwz=(Lf*(Fx(1)*sin(detal)+Fy(1)*cos(detal))-0.5*Bf*(Fx(1)*cos(detal)-Fy(1)*sin(detal)))/Iz+(Lf*(Fx(2)*sin(detar)+Fy(2)*cos(detar))+0.5*Bf*(Fx(2)*cos(detar)-Fy(2)*sin(detar)))/Iz-(0.5*Br*Fx(3)+Lr*Fy(3))/Iz+(0.5*Br*Fx(4)-Lr*Fy(4))/Iz;
end

== matlab function Dugoff0407/实际力输入估计单个miu ==
  data: Fxfl input; x0 output; Fxfr input; Fxrl input; Fxrr input; Fyfl input; Fyfr input; Fyrl input; Fyrr input; ax input; ay input; dwz input; deta input; detar input
function x0 = fcn(Fxfl,Fxfr,Fxrl,Fxrr,Fyfl,Fyfr,Fyrl,Fyrr,ax,ay,dwz,deta,detar)
persistent X P;
if isempty(X)
    X = 0.6;
    P =0.001;
end

m=1412;
la=1.015; %质心距离前轴的距离m 1.27 
lb=1.895; %质心距离后轴的距离m
Tf=1.675; %前轴轮距m
Tr=1.675; %后轴轮距m 1.55
Iz=1536.7; %整车z轴转动惯量kg*m^2
Q = 0.001;
R = diag([1,1,1])*50;
Xpre = X;
%F = diag([1,1,1,1]);
H = [(Fxfl*cos(deta)-Fyfl*sin(deta))/m+(Fxfr*cos(detar)-Fyfr*sin(detar))/m+Fxrl/m+Fxrr/m;(Fxfl*sin(deta)+Fyfl*cos(deta))/m+(Fxfr*sin(detar)+Fyfr*cos(deta))/m+Fyrl/m+Fyrr/m;(la*(Fxfl*sin(deta)+Fyfl*cos(deta))-Tf/2*(Fxfl*cos(deta)-Fyfl*sin(deta)))/Iz+(la*(Fxfr*sin(detar)+Fyfr*cos(detar))+Tf/2*(Fxfr*cos(detar)-Fyfr*sin(detar)))/Iz+(-Tr/2*Fxrl-lb*Fyrl)/Iz+(Tr/2*Fxrr-lb*Fyrr)/Iz];
zjian =H*Xpre; 
PP=P+Q;
% if a>0
if (H*PP*H')~=zeros(3,3)

% if(det(H*PP*H'+R)==0)
%     X = ones(4, 1);
% else
Kk=PP*H'/(H*PP*H'+R);
X=Xpre+Kk*([ax,ay,dwz]'-zjian);
P=PP-Kk*H*PP;
% end
% 
% if(X(1)>1||X(1)<0||X(2)<0||X(3)<0||X(4)<0||X(2)>1||X(3)>1||X(4)>1)
%     X=0.8;
%     P=0.001;
% else
% end
x0=X;
else
    x0 = zeros(1,1);
    
end
% else
%     x0 = zeros(4,1);
%     X=ones(4, 1)*0.5;
%     P=diag([1,1,1,1])*0.1;
%     ccc = 2;
% end
end

== matlab function Dugoff0407/MATLAB Function ==
  data: ddxh input; x0 output; dtheta input; xh input; theta input; ax input
function x0 = fcn(ddxh,dtheta,xh,theta,ax)
persistent X P;
if isempty(X)
    X = ones(10,1)*0.001;
    P =diag(ones(1,10));
end
dt=0.01;
%mh=730;
%Iy=1200;
%mf=55;
%mr=52.5;
%kf=28.6;
%kr=39.6;
%cf=1.85;
%cr=1.5;
%ktf=247.03;
%ktr=247.03;
%lf=1.187;
%lr=1.533;
%h=0.6;


mh=1270;
Iy=1536.7;
mf=71;
mr=71;
kf=27*1000;
kr=30*1000;
cf=1.85*1000;
cr=1.5*1000;
ktf=268*1000;
ktr=268*1000;
lf=1.015;
lr=1.895;
h=0.54;
M=diag([mh,Iy,mf,mr]);
C=[cf+cr,-cf*lf+cr*lr,-cf,-cr;
    -lf*cf+lr*cr,lf*lf*cf+lr*lr*cr,+lf*cf,-lr*cr;
    -cf,+lf*cf,cf,0;
    -cr,-lr*cr,0,cr];
K=[kf+kr,-kf*lf+kr*lr,-kf,-kr;
    -lf*kf+lr*kr,lf*lf*kf+lr*lr*kr,+lf*kf,-lr*kr;
    -kf,+kf*lf,ktf+kf,0;
    -kr,-kr*lr,0,ktr+kr];
F=[0,mh*h,0,0]';F1=[0,0;0,0;ktf,0;0,ktr];A=[zeros(4,4),eye(4);-M^(-1)*K,-M^(-1)*C];B=[zeros(4,1);M^(-1)*F];
B1=[zeros(4,2);M^(-1)*F1];
Aa=[A ,B1;zeros(2,8),zeros(2,2)];Ba=[B;zeros(2,1)];
H=[-K(1,:),-C(1,:);zeros(1,4),0,1,0,0;1,zeros(1,7);0,1,zeros(1,6)];
Hd=[H,zeros(4,2)];
coder.extrinsic('c2d');
Ad=zeros(10,10);Bd=zeros(10,1);
[Ad,Bd]=c2d(Aa,Ba,dt);

Qa=diag([ones(1,4)*10^(-7),ones(1,4)*10^(-4),0.00001,0.00001])*1000;
R=diag(ones(1,4))*0.0000001;

Xpre=X;
Xpd=Ad*Xpre+Bd*ax;
Ppd=Ad*P*Ad'+Qa;
K=Ppd*Hd'*(Hd*Ppd*Hd'+R)^(-1);
X=Xpd+K*([ddxh,dtheta,xh,theta]'-Hd*Xpd);
P=(eye(10)-K*Hd)*Ppd;
x0=X;
end

== matlab function Dugoff0407/Dugoff轮胎模型/tyre11 ==
  data: Fx11 output; Fy11 output; Fz11 input; alpha11 input; lamda11 input; mu input
function [Fx11,Fy11] = fcn(Fz11,alpha11,lamda11,mu)
lamda11=-lamda11;

  Cx=-30; 
  Cy=-18;    

S=(1-lamda11)/(2*sqrt((Cx^2)*(lamda11^2)+(Cy^2)*(tan(alpha11))^2));
if S<1
   f=S*(2-S);
else            %S>=1
   f=1;
end


Fx11=Fz11*mu*Cx*lamda11*f/(1-lamda11);
Fy11=Fz11*mu*Cy*tan(alpha11)*f/(1-lamda11);
% 
%   Cx=-30; 
%   Cy=-18;

== matlab function Dugoff0407/Dugoff轮胎模型/tyre12 ==
  data: Fx12 output; Fy12 output; Fz12 input; alpha12 input; lamda12 input; mu input
function [Fx12,Fy12] = fcn(Fz12,alpha12,lamda12,mu)
lamda12=-lamda12;

 Cx=-28;
 Cy=-18.5;

S=(1-lamda12)/(2*sqrt(Cx^2*lamda12^2+Cy^2*(tan(alpha12))^2));
if S<1
   f=S*(2-S);
else
   f=1;
end
Fx12=Fz12*mu*Cx*lamda12*f/(1-lamda12);
Fy12=Fz12*mu*Cy*tan(alpha12)*f/(1-lamda12);


%  Cx=-28;
%  Cy=-18.5;

== matlab function Dugoff0407/Dugoff轮胎模型/tyre21 ==
  data: Fx21 output; Fy21 output; Fz21 input; alpha21 input; lamda21 input; mu input
function [Fx21,Fy21] = fcn(Fz21,alpha21,lamda21,mu)
lamda21=-lamda21

  Cx=-30;
  Cy=-20.5;

S=(1-lamda21)/(2*sqrt((Cx^2)*(lamda21^2)+(Cy^2)*((tan(alpha21))^2)));
if S<1
   f=S*(2-S);
else
   f=1;
end
Fx21=Fz21*mu*Cx*lamda21*f/(1-lamda21);
Fy21=Fz21*mu*Cy*tan(alpha21)*f/(1-lamda21);

%   Cx=-30;
%   Cy=-20.5;

== matlab function Dugoff0407/Dugoff轮胎模型/tyre22 ==
  data: Fx22 output; Fy22 output; Fz22 input; alpha22 input; lamda22 input; mu input
function [Fx22,Fy22] = fcn(Fz22,alpha22,lamda22,mu)
  lamda22=-lamda22
  
  Cx=-31;
  Cy=-20;

S=(1-lamda22)/(2*sqrt(Cx^2*lamda22^2+Cy^2*(tan(alpha22))^2));
if S<1
   f=S*(2-S);
else
   f=1;
end
Fx22=Fz22*mu*Cx*lamda22*f/(1-lamda22);
Fy22=Fz22*mu*Cy*tan(alpha22)*f/(1-lamda22);

%   Cx=-31;
%   Cy=-20;
